simulink model "blink_exec"  (Simulink 3.00)
libraries: execlib x5

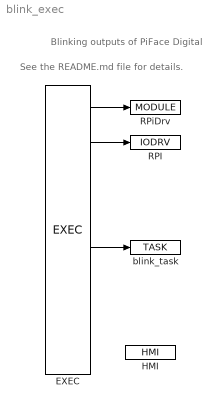
== system blink_exec ==
  note: See the README.md file for details.
  note: Blinking outputs of PiFace Digital
  EXEC : execlib/EXEC  target=PC - Linux  tick=0.02  ntick0=1  ntick1=50  ntick2=100  ntick3=1200  pri0=5  pri1=9  pri2=13  pri3=18
  HMI : execlib/HMI  IncludeHMI=on  HmiDir=hmi  SourceDir=hmisrc  GenerateWebWatch=on  GenerateRexHMI=on  RedirectToHMI=off  Compression=off
  RPI : execlib/IODRV  module=RPiDrv  classname=RPiDrv  factor=1  stack=10240  pri=3  timer=off
  RPiDrv : execlib/MODULE
  blink_task : execlib/TASK  factor=1  start=0  stop=1  stack=10240  MDLOPEN=on
  wires:
  EXEC/1 -> RPiDrv/1
  EXEC/2 -> RPI/1
  EXEC/5 -> blink_task/1
